simulink model "controller_position"  (R2021a)
settings: Solver=FixedStepAuto  StartTime=0.0  StopTime=10.0  FixedStep=0.002  RelTol=1e-3
undefined symbols (not defined in the file): Ts_pos_control
settings Model: Creator=francois  LastModifiedBy=esl
settings SolverCC: AlgebraicLoopSolver=TrustRegion
settings DebuggingCC: ModelReferenceExtraNoncontSigs=none  SFMachineParentedDataDiag=warning

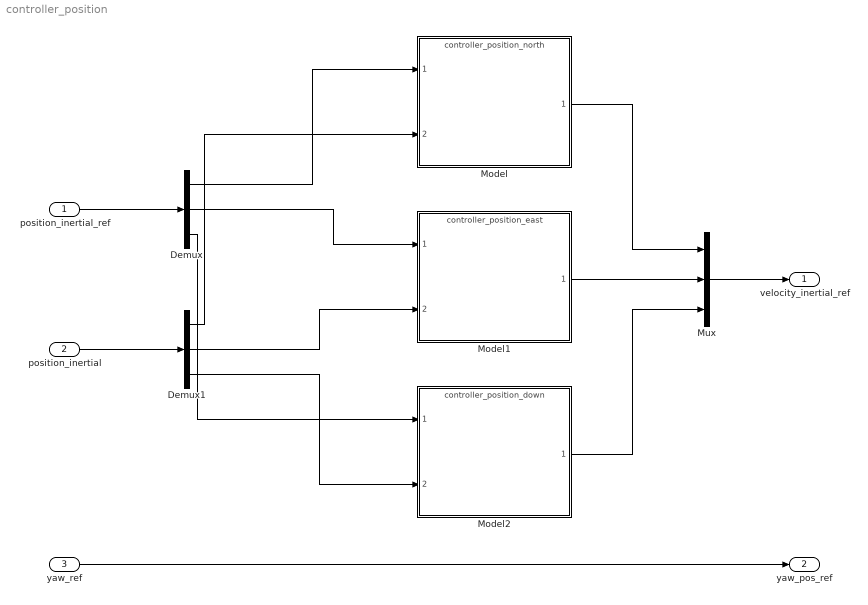
== system controller_position ==
  position_inertial_ref : Inport  SampleTime=Ts_pos_control
  position_inertial : Inport  Port=2  SampleTime=Ts_pos_control
  yaw_ref : Inport  Port=3  SampleTime=Ts_pos_control
  Demux : Demux  Outputs=3
  Demux1 : Demux  Outputs=3
  Model : ModelReference  ModelNameDialog=controller_position_north.slx  SimulationMode=Normal  ModelReferenceVersion=3.14
  Model1 : ModelReference  ModelNameDialog=controller_position_east.slx  SimulationMode=Normal  ModelReferenceVersion=3.12
  Model2 : ModelReference  ModelNameDialog=controller_position_down.slx  SimulationMode=Normal  ModelReferenceVersion=3.13
  Mux : Mux  Inputs=3
  velocity_inertial_ref : Outport  SampleTime=Ts_pos_control
  yaw_pos_ref : Outport  Port=2  SampleTime=Ts_pos_control  VectorParamsAs1DForOutWhenUnconnected=off
  wires:
  Model/1 -> Mux/1
  Model1/1 -> Mux/2
  Model2/1 -> Mux/3
  Mux/1 -> velocity_inertial_ref/1
  position_inertial/1 -> Demux1/1
  position_inertial_ref/1 -> Demux/1
  Demux/1 -> Model/1
  Demux1/1 -> Model/2
  Demux/2 -> Model1/1
  Demux1/3 -> Model2/2
  Demux/3 -> Model2/1
  Demux1/2 -> Model1/2
  yaw_ref/1 -> yaw_pos_ref/1
